simulink model "q4_ode_filter"  (R2020b)
settings: Solver=ode45  StartTime=0.0  StopTime=15.0  RelTol=1e-3
values from neighbouring files (symbols this model uses):
  CCF = R(ndof+1:ntot,1:ndof)    [M4_script.m]
  CFF = R(1:ndof,1:ndof)    [M4_script.m]
  extract_ya = zeros(ndof,1); extract_ya(dof_ya)=1    [M4_script.m]
  KCF = K(ndof+1:ntot,1:ndof)    [M4_script.m]
  KFF = K(1:ndof,1:ndof)    [M4_script.m]
  MCF = M(ndof+1:ntot,1:ndof)    [M4_script.m]
  MFF = M(1:ndof,1:ndof)    [M4_script.m]
  ndof = 153    [M4_script.m]
libraries: cstblocks x2
settings Model: Creator=Gianciccetto  LastModifiedBy=Gianciccetto

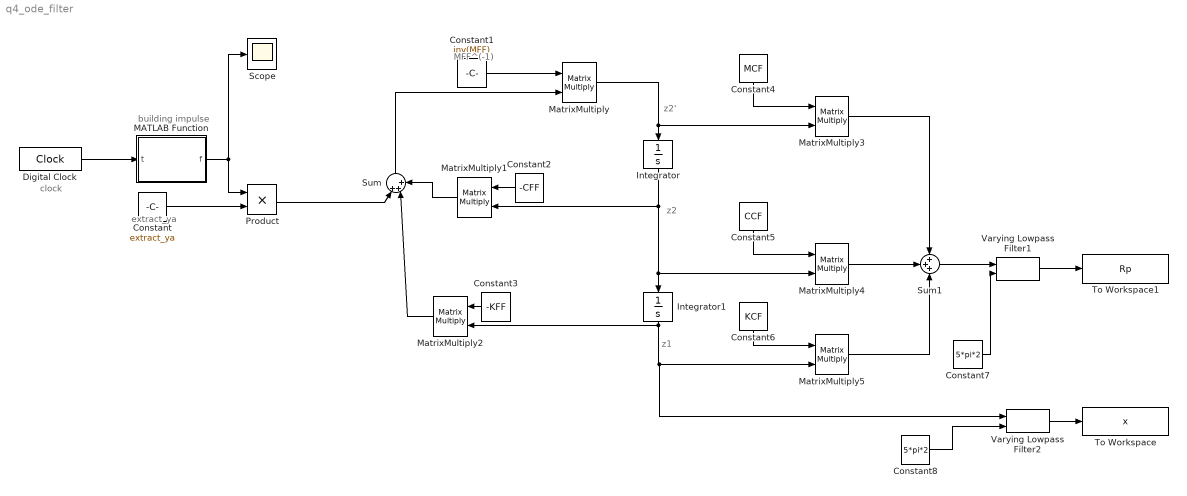
== system q4_ode_filter ==
  note: building impulse
  note: clock
  note: extract_ya
  note: MFF^(-1)
  note: z1
  note: z2
  note: z2'
  Constant : Constant  Value=extract_ya
  Constant1 : Constant  Value=inv(MFF)
  Constant2 : Constant  Value=-CFF
  Constant3 : Constant  Value=-KFF
  Constant4 : Constant  Value=MCF
  Constant5 : Constant  Value=CCF
  Constant6 : Constant  Value=KCF
  Constant7 : Constant  Value=5*pi*2
  Constant8 : Constant  Value=5*pi*2
  Digital Clock : DigitalClock  SampleTime=0.0001
  Integrator : Integrator  InitialCondition=zeros(ndof,1)
  Integrator1 : Integrator  InitialCondition=zeros(ndof,1)
  MATLAB Function : MATLAB Function  TreatAsAtomicUnit=on
  MatrixMultiply{,1..5} (6 alike) : Product  Multiplication=Matrix(*)
  Product : Product
  Scope : Scope
  Sum : Sum  Inputs=|+++
  Sum1 : Sum  Inputs=+++
  To Workspace : ToWorkspace  VariableName=x  SampleTime=-1
  To Workspace1 : ToWorkspace  VariableName=Rp  SampleTime=-1
  Varying Lowpass Filter1 : cstblocks/Linear Parameter Varying/Varying Lowpass Filter  N=20
  Varying Lowpass Filter2 : cstblocks/Linear Parameter Varying/Varying Lowpass Filter  N=20
  wires:
  MATLAB Function/1(f) -> Product/1, Scope/1
  Digital Clock/1 -> MATLAB Function/1(t)
  Constant/1 -> Product/2
  Constant1/1 -> MatrixMultiply/1
  Sum/1 -> MatrixMultiply/2
  MatrixMultiply/1 -> MatrixMultiply3/2, Integrator/1
  Integrator/1 -> MatrixMultiply4/2, Integrator1/1, MatrixMultiply1/2
  Integrator1/1 -> MatrixMultiply2/2, Varying Lowpass Filter2/1, MatrixMultiply5/2
  Constant2/1 -> MatrixMultiply1/1
  Constant3/1 -> MatrixMultiply2/1
  MatrixMultiply1/1 -> Sum/3
  MatrixMultiply2/1 -> Sum/2
  Constant4/1 -> MatrixMultiply3/1
  Constant5/1 -> MatrixMultiply4/1
  Constant6/1 -> MatrixMultiply5/1
  MatrixMultiply4/1 -> Sum1/2
  MatrixMultiply3/1 -> Sum1/1
  MatrixMultiply5/1 -> Sum1/3
  Sum1/1 -> Varying Lowpass Filter1/1
  Product/1 -> Sum/1
  Constant7/1 -> Varying Lowpass Filter1/2
  Varying Lowpass Filter1/1 -> To Workspace1/1
  Varying Lowpass Filter2/1 -> To Workspace/1
  Constant8/1 -> Varying Lowpass Filter2/2

== matlab function q4_ode_filter/MATLAB Function ==
  data: t input; f output
function f = fcn(t)
%% Impulse (half-sine) definition


Fmax=4000;
Ti=2*0.3; % period of the half-sine function
fi=1/Ti; % freq. of the half-sine function
f=zeros(size(t));
for j=1:length(t)
    if t(j)<=0.3
        f(j)=Fmax*sin(2*pi*fi*t(j));
    else
        f(j)=0;
    end
   
end
